simulink model "sil_test"  (R2022b)
settings: Solver=VariableStepAuto  StartTime=0.0  StopTime=inf  RelTol=1e-3
undefined symbols (not defined in the file): battery_monitor, battery_monitor_lib, BM_STATUSES, canChannel, DI_STATUSES, driver_interface, driver_interface_lib, Ended, governor, governor_lib, MI_STATUSES, motor_interface, motor_interface_lib, simp_vd_interface, simp_vd_lib, Single
libraries: canmsglib x16, canlib x10, simulink x6, speedgoatlib_IO191 x5, slrealtimeiplib x3, AMK_comms_plant_lib x1, BMS_plant_lib x1, speedgoatlib_IO614 x1, slrealtimeutilitieslib x1, etargetslib x1
(part 2 of 3)

== system sil_test/Function-Call Subsystem ==
  In1 : Inport
  function : TriggerPort  TriggerType=function-call  VariantControl=(inherit)
  Bus Creator : BusCreator  Inputs=2
  Bus Creator1 : BusCreator  Inputs=7
  Bus Creator2 : BusCreator  Inputs=7
  CAN Unpack : canmsglib/CAN Unpack  CANdbFile=C:\Users\LinF\Documents\MACFE\Embedded\CAN_Stuff\CAN_Databases\CAN_AMKInverter.dbc  MsgList=AMK0_SetPoints1  MsgName=AMK0_SetPoints1  MsgIDType=Standard (11-bit identifier)  MsgIdentifier=389  MsgLength=8  SignalInfo={'AMK_TargetVelocity','16','16','LE','signed','Standard','0','1','0','-Inf','Inf';'AMK_TorqueLimitNegativ','48','16','LE','signed','Standard','0','1','0','-Inf','Inf';'AMK_TorqueLimitPositiv','32','16','LE','signed','Standard','0','1','0','-Inf','Inf';'AMK_bDcOn','9','1','LE','unsigned','Standard','0','1','0','-Inf','Inf';'AMK_bEnable','10','1','LE','unsigned','Standard','0','1','0','-Inf','Inf';'AMK_bErrorReset','11','1','LE','unsigned','Standard','0','1','0','-Inf','Inf';'AMK_bInverterOn','8','1','LE','unsigned','Standard','0','1','0','-Inf','Inf'}  IDPort=off  TimestampPort=off  ErrorPort=off  RemotePort=off  LengthPort=off  StatusPort=off  ApplyMinMax=off
      settings: LibrarySourceBlock=canlib/CAN Unpack  DataFormat=CANdb specified signals
  CAN Unpack1 : canmsglib/CAN Unpack  CANdbFile=C:\Users\LinF\Documents\MACFE\Embedded\CAN_Stuff\CAN_Databases\CAN_AMKInverter.dbc  MsgList=AMK1_SetPoints1  MsgName=AMK1_SetPoints1  MsgIDType=Standard (11-bit identifier)  MsgIdentifier=390  MsgLength=8  SignalInfo={'AMK_TargetVelocity','16','16','LE','signed','Standard','0','1','0','-Inf','Inf';'AMK_TorqueLimitNegativ','48','16','LE','signed','Standard','0','1','0','-Inf','Inf';'AMK_TorqueLimitPositiv','32','16','LE','signed','Standard','0','1','0','-Inf','Inf';'AMK_bDcOn','9','1','LE','unsigned','Standard','0','1','0','-Inf','Inf';'AMK_bEnable','10','1','LE','unsigned','Standard','0','1','0','-Inf','Inf';'AMK_bErrorReset','11','1','LE','unsigned','Standard','0','1','0','-Inf','Inf';'AMK_bInverterOn','8','1','LE','unsigned','Standard','0','1','0','-Inf','Inf'}  IDPort=off  TimestampPort=off  ErrorPort=off  RemotePort=off  LengthPort=off  StatusPort=off  ApplyMinMax=off
      settings: LibrarySourceBlock=canlib/CAN Unpack  DataFormat=CANdb specified signals
  pt_CAN_IN : Outport
  wires:
  Bus Creator/1 -> pt_CAN_IN/1
  Bus Creator2/1 -> Bus Creator/2  "ptCAN_AMK1_Setpoints1_Right"
  Bus Creator1/1 -> Bus Creator/1  "ptCAN_AMK0_Setpoints1_Left"
  In1/1 -> CAN Unpack/1, CAN Unpack1/1
  CAN Unpack/1 -> Bus Creator1/1  "AMK0_TargetVelocity"
  CAN Unpack/2 -> Bus Creator1/2  "AMK0_TorqueLimitNegativ"
  CAN Unpack/3 -> Bus Creator1/3  "AMK0_TorqueLimitPositiv"
  CAN Unpack/4 -> Bus Creator1/4  "AMK0_bDcOn"
  CAN Unpack/5 -> Bus Creator1/5  "AMK0_bEnable"
  CAN Unpack/6 -> Bus Creator1/6  "AMK0_bErrorReset"
  CAN Unpack/7 -> Bus Creator1/7  "AMK0_bInverterOn"
  CAN Unpack1/3 -> Bus Creator2/3  "AMK1_TorqueLimitPositiv"
  CAN Unpack1/6 -> Bus Creator2/6  "AMK1_bErrorReset"
  CAN Unpack1/4 -> Bus Creator2/4  "AMK1_bDcOn"
  CAN Unpack1/7 -> Bus Creator2/7  "AMK1_bInverterOn"
  CAN Unpack1/2 -> Bus Creator2/2  "AMK1_TorqueLimitNegativ"
  CAN Unpack1/5 -> Bus Creator2/5  "AMK1_bEnable"
  CAN Unpack1/1 -> Bus Creator2/1  "AMK1_TargetVelocity"

== system sil_test/Function-Call Subsystem1 ==
  In1 : Inport
  function : TriggerPort  TriggerType=function-call  VariantControl=(inherit)
  Bus Creator1 : BusCreator  Inputs=3
  CAN Unpack : canmsglib/CAN Unpack  CANdbFile=C:\Users\LinF\Documents\MACFE\Controls\repos\can_dbc\dbcs\VEH_CAN.dbc  MsgList=Contactor_States  MsgName=Contactor_States  MsgIDType=Standard (11-bit identifier)  MsgIdentifier=1570  MsgLength=3  SignalInfo={'Pack_Negative','16','8','LE','unsigned','Standard','0','1','0','-Inf','Inf';'Pack_Positive','0','8','LE','unsigned','Standard','0','1','0','-Inf','Inf';'Pack_Precharge','8','8','LE','unsigned','Standard','0','1','0','-Inf','Inf'}  IDPort=off  TimestampPort=off  ErrorPort=off  RemotePort=off  LengthPort=off  StatusPort=off  ApplyMinMax=off
      settings: LibrarySourceBlock=canlib/CAN Unpack  DataFormat=CANdb specified signals
  pt_CAN_IN : Outport
  wires:
  Bus Creator1/1 -> pt_CAN_IN/1  "ptCAN_AMK_Setpoints1_Left"
  In1/1 -> CAN Unpack/1
  CAN Unpack/3 -> Bus Creator1/3  "precharge"
  CAN Unpack/1 -> Bus Creator1/1  "AIR_neg"
  CAN Unpack/2 -> Bus Creator1/2  "AIR_pos"

== system sil_test/Function-Call Subsystem2 ==
  In1 : Inport
  function : TriggerPort  TriggerType=function-call  VariantControl=(inherit)
  CAN Unpack : canmsglib/CAN Unpack  CANdbFile=C:\Users\maxfa\OneDrive\Documents\vehicle_control_system\src\testing\Vehicle_HIL_plant\VEH_CAN.dbc  MsgList=Contactor_Feedback  MsgName=Contactor_Feedback  MsgIDType=Standard (11-bit identifier)  MsgIdentifier=1574  MsgLength=3  SignalInfo={'Pack_Negative_Feedback','8','1','LE','unsigned','Standard','0','1','0','0','1';'Pack_Positive_Feedback','0','1','LE','unsigned','Standard','0','1','0','0','1';'Pack_Precharge_Feedback','16','1','LE','unsigned','Standard','0','1','0','0','1'}  IDPort=off  TimestampPort=off  ErrorPort=off  RemotePort=off  LengthPort=off  StatusPort=off  ApplyMinMax=off
      settings: LibrarySourceBlock=canlib/CAN Unpack  DataFormat=CANdb specified signals
  BM_b_prechrgContactorSts : Outport
  BM_b_HVposContactorSts : Outport  Port=2
  BM_b_HVnegContactorSts : Outport  Port=3
  wires:
  In1/1 -> CAN Unpack/1
  CAN Unpack/1 -> BM_b_HVnegContactorSts/1
  CAN Unpack/3 -> BM_b_prechrgContactorSts/1
  CAN Unpack/2 -> BM_b_HVposContactorSts/1

== system sil_test/Speedgoat Inputs ==
  "Analog input " : speedgoatlib_IO191/Analog input   parModuleId=1  parSampleTime=-1  parPciSlot=-1  parAdcChannels=[1 2 3 4 5 6 7 8]  parAdcMode=2  parAdcRanges=[4 4 4 4 4 4 4 4]  parAdcInitValues=[0 0]  parAdcResets=[1 1]  paramsAdcDma=[0 1 200 -1]
      settings: SourceProductName=Simulink Real-Time: Speedgoat I/O Blockset
  Bus Creator : BusCreator  Inputs=16
  "Digital input " : speedgoatlib_IO191/Digital input   parModuleId=1  parSampleTime=-1  parPciSlot=-1  parDiChannels=[1 2 3 4 5 6 7 8]
      settings: SourceProductName=Simulink Real-Time: Speedgoat I/O Blockset
  Speedgoat Inputs : Outport
  inverter_en : Outport  Port=2
  wires:
  Bus Creator/1 -> Speedgoat Inputs/1
  "Digital input "/1 -> inverter_en/1, Bus Creator/1  "DIO1"
  "Digital input "/2 -> Bus Creator/2  "DIO2"
  "Digital input "/3 -> Bus Creator/3  "DIO3"
  "Digital input "/4 -> Bus Creator/4  "DIO4"
  "Digital input "/5 -> Bus Creator/5  "DIO5"
  "Digital input "/6 -> Bus Creator/6  "DIO6"
  "Digital input "/7 -> Bus Creator/7  "DIO7"
  "Digital input "/8 -> Bus Creator/8  "DIO8"
  "Analog input "/1 -> Bus Creator/9  "AI1"
  "Analog input "/2 -> Bus Creator/10  "AI2"
  "Analog input "/3 -> Bus Creator/11  "AI3"
  "Analog input "/4 -> Bus Creator/12  "AI4"
  "Analog input "/5 -> Bus Creator/13  "AI5"
  "Analog input "/6 -> Bus Creator/14  "AI6"
  "Analog input "/7 -> Bus Creator/15  "AI7"
  "Analog input "/8 -> Bus Creator/16  "AI8"

== system sil_test/Speedgoat Outputs ==
  Speedgoat Outputs : Inport
  "Analog output " : speedgoatlib_IO191/Analog output   parModuleId=1  parSampleTime=-1  parPciSlot=-1  parDacChannels=[1 2 3 4]  parModuleType=1  parDacRanges=[3 3 3 3]  parDacInitValues=[0 0 0 0]  parDacResets=[1 1 1 1]
      settings: SourceProductName=Simulink Real-Time: Speedgoat I/O Blockset
  Bus Selector : BusSelector  OutputSignals=DO9,DO10,DO11,DO12,DO13,DO14,DO15,DO16,AO1,AO2,AO3,AO4
  "Digital output " : speedgoatlib_IO191/Digital output   parModuleId=1  parSampleTime=-1  parPciSlot=-1  parDoChannels=[9 10 11 12 13 14 15 16]  parDoInitValues=[0 0 0 0 0 0 0 0]  parDoResets=[1 1 1 1 1 1 1 1]
      settings: SourceProductName=Simulink Real-Time: Speedgoat I/O Blockset
  wires:
  Speedgoat Outputs/1 -> Bus Selector/1
  Bus Selector/4 -> "Digital output "/4  "<DO12>"
  Bus Selector/1 -> "Digital output "/1  "<DO9>"
  Bus Selector/2 -> "Digital output "/2  "<DO10>"
  Bus Selector/5 -> "Digital output "/5  "<DO13>"
  Bus Selector/3 -> "Digital output "/3  "<DO11>"
  Bus Selector/6 -> "Digital output "/6  "<DO14>"
  Bus Selector/7 -> "Digital output "/7  "<DO15>"
  Bus Selector/8 -> "Digital output "/8  "<DO16>"
  Bus Selector/9 -> "Analog output "/1  "<AO1>"
  Bus Selector/10 -> "Analog output "/2  "<AO2>"
  Bus Selector/11 -> "Analog output "/3  "<AO3>"
  Bus Selector/12 -> "Analog output "/4  "<AO4>"

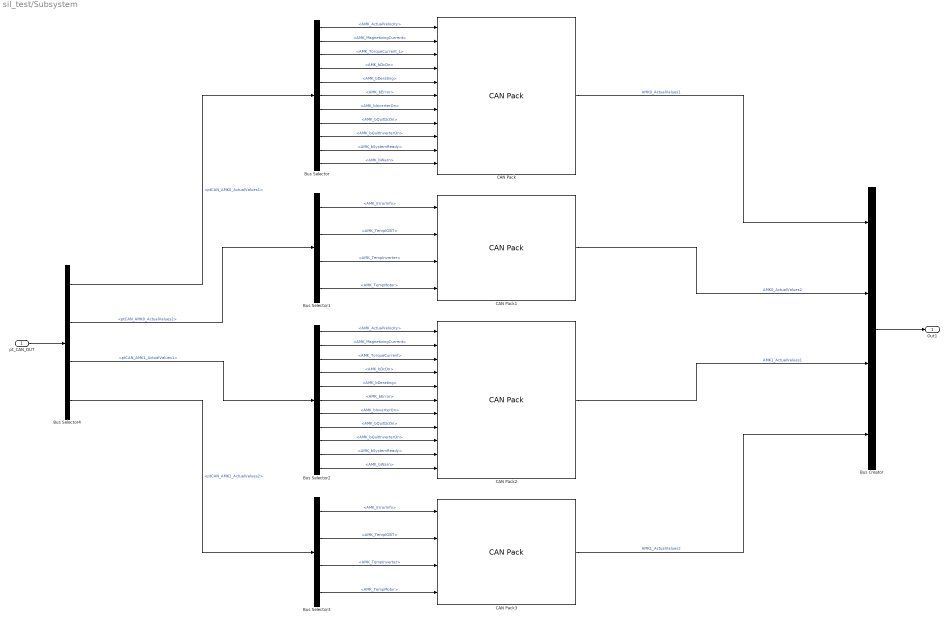
== system sil_test/Subsystem ==
  pt_CAN_OUT : Inport
  Bus Creator : BusCreator  Inputs=4
  Bus Selector : BusSelector  OutputSignals=AMK_ActualVelocity,AMK_MagnetizingCurrent,AMK_TorqueCurrent_L,AMK_bDcOn,AMK_bDerating,AMK_bError,AMK_bInverterOn,AMK_bQuitDcOn,AMK_bQuitInverterOn,AMK_bSystemReady,AMK_bWarn
  Bus Selector1 : BusSelector  OutputSignals=AMK_ErrorInfo,AMK_TempIGBT,AMK_TempInverter,AMK_TempMotor
  Bus Selector2 : BusSelector  OutputSignals=AMK_ActualVelocity,AMK_MagnetizingCurrent,AMK_TorqueCurrent,AMK_bDcOn,AMK_bDerating,AMK_bError,AMK_bInverterOn,AMK_bQuitDcOn,AMK_bQuitInverterOn,AMK_bSystemReady,AMK_bWarn
  Bus Selector3 : BusSelector  OutputSignals=AMK_ErrorInfo,AMK_TempIGBT,AMK_TempInverter,AMK_TempMotor
  Bus Selector4 : BusSelector  OutputSignals=ptCAN_AMK0_ActualValues1,ptCAN_AMK0_ActualValues2,ptCAN_AMK1_ActualValues1,ptCAN_AMK1_ActualValues2
  CAN Pack : canmsglib/CAN Pack  CANdbFile=C:\Users\LinF\Documents\MACFE\Embedded\CAN_Stuff\CAN_Databases\CAN_AMKInverter.dbc  MsgList=AMK0_ActualValues1  MsgName=AMK0_ActualValues1  MsgIDType=Standard (11-bit identifier)  MsgIdentifier=644  MsgLength=8  Remote=off  ApplyMinMax=off  BusOutput=off  SignalInfo={'AMK_ActualVelocity','16','16','LE','signed','Standard','0','1','0','-Inf','Inf';'AMK_MagnetizingCurrent','48','16','LE','signed','Standard','0','1','0','-Inf','Inf';'AMK_TorqueCurrent','32','16','LE','signed','Standard','0','1','0','-Inf','Inf';'AMK_bDcOn','12','1','LE','unsigned','Standard','0','1','0','-Inf','Inf';'AMK_bDerating','15','1','LE','unsigned','Standard','0','1','0','-Inf','Inf';'AMK_bError','9','1','LE','unsigned','Standard','0','1','0','-Inf','Inf';'AMK_bInverterOn','14','1','LE','unsigned','Standard','0','1','0','-Inf','Inf';'AMK_bQuitDcOn','11','1','LE','unsigned','Standard','0','1','0','-Inf','Inf';'AMK_bQuitInverterOn','13','1','LE','unsigned','Standard','0','1','0','-Inf','Inf';'AMK_bSystemReady','8','1','LE','unsigned','Standard','0','1','0','-Inf','Inf';'AMK_bWarn','10','1','LE','unsigned','Standard','0','1','0','-Inf','Inf'}
      settings: LibrarySourceBlock=canlib/CAN Pack  DataFormat=CANdb specified signals
  CAN Pack1 : canmsglib/CAN Pack  CANdbFile=C:\Users\LinF\Documents\MACFE\Embedded\CAN_Stuff\CAN_Databases\CAN_AMKInverter.dbc  MsgList=AMK0_ActualValues2  MsgName=AMK0_ActualValues2  MsgIDType=Standard (11-bit identifier)  MsgIdentifier=646  MsgLength=8  Remote=off  ApplyMinMax=off  BusOutput=off  SignalInfo={'AMK_ErrorInfo','32','16','LE','unsigned','Standard','0','1','0','0','65535';'AMK_TempIGBT','48','16','LE','signed','Standard','0','0.1','0','-3276.8','3276.7';'AMK_TempInverter','16','16','LE','signed','Standard','0','0.1','0','-3276.8','3276.7';'AMK_TempMotor','0','16','LE','signed','Standard','0','0.1','0','-3276.8','3276.7'}
      settings: LibrarySourceBlock=canlib/CAN Pack  DataFormat=CANdb specified signals
  CAN Pack2 : canmsglib/CAN Pack  CANdbFile=C:\Users\LinF\Documents\MACFE\Embedded\CAN_Stuff\CAN_Databases\CAN_AMKInverter.dbc  MsgList=AMK1_ActualValues1  MsgName=AMK1_ActualValues1  MsgIDType=Standard (11-bit identifier)  MsgIdentifier=645  MsgLength=8  Remote=off  ApplyMinMax=off  BusOutput=off  SignalInfo={'AMK_ActualVelocity','16','16','LE','signed','Standard','0','1','0','-Inf','Inf';'AMK_MagnetizingCurrent','48','16','LE','signed','Standard','0','1','0','-Inf','Inf';'AMK_TorqueCurrent','32','16','LE','signed','Standard','0','1','0','-Inf','Inf';'AMK_bDcOn','12','1','LE','unsigned','Standard','0','1','0','-Inf','Inf';'AMK_bDerating','15','1','LE','unsigned','Standard','0','1','0','-Inf','Inf';'AMK_bError','9','1','LE','unsigned','Standard','0','1','0','-Inf','Inf';'AMK_bInverterOn','14','1','LE','unsigned','Standard','0','1','0','-Inf','Inf';'AMK_bQuitDcOn','11','1','LE','unsigned','Standard','0','1','0','-Inf','Inf';'AMK_bQuitInverterOn','13','1','LE','unsigned','Standard','0','1','0','-Inf','Inf';'AMK_bSystemReady','8','1','LE','unsigned','Standard','0','1','0','-Inf','Inf';'AMK_bWarn','10','1','LE','unsigned','Standard','0','1','0','-Inf','Inf'}
      settings: LibrarySourceBlock=canlib/CAN Pack  DataFormat=CANdb specified signals
  CAN Pack3 : canmsglib/CAN Pack  CANdbFile=C:\Users\LinF\Documents\MACFE\Embedded\CAN_Stuff\CAN_Databases\CAN_AMKInverter.dbc  MsgList=AMK1_ActualValues2  MsgName=AMK1_ActualValues2  MsgIDType=Standard (11-bit identifier)  MsgIdentifier=647  MsgLength=8  Remote=off  ApplyMinMax=off  BusOutput=off  SignalInfo={'AMK_ErrorInfo','32','16','LE','unsigned','Standard','0','1','0','0','65535';'AMK_TempIGBT','48','16','LE','signed','Standard','0','0.1','0','-3276.8','3276.7';'AMK_TempInverter','16','16','LE','signed','Standard','0','0.1','0','-3276.8','3276.7';'AMK_TempMotor','0','16','LE','signed','Standard','0','0.1','0','-3276.8','3276.7'}
      settings: LibrarySourceBlock=canlib/CAN Pack  DataFormat=CANdb specified signals
  Out1 : Outport
  wires:
  CAN Pack/1 -> Bus Creator/1  "AMK0_ActualValues1"
  CAN Pack1/1 -> Bus Creator/2  "AMK0_ActualValues2"
  CAN Pack2/1 -> Bus Creator/3  "AMK1_ActualValues1"
  CAN Pack3/1 -> Bus Creator/4  "AMK1_ActualValues2"
  Bus Selector4/1 -> Bus Selector/1  "<ptCAN_AMK0_ActualValues1>"
  Bus Selector4/2 -> Bus Selector1/1  "<ptCAN_AMK0_ActualValues2>"
  Bus Selector4/3 -> Bus Selector2/1  "<ptCAN_AMK1_ActualValues1>"
  Bus Selector4/4 -> Bus Selector3/1  "<ptCAN_AMK1_ActualValues2>"
  pt_CAN_OUT/1 -> Bus Selector4/1
  Bus Creator/1 -> Out1/1
  Bus Selector/1 -> CAN Pack/1  "<AMK_ActualVelocity>"
  Bus Selector/3 -> CAN Pack/3  "<AMK_TorqueCurrent_L>"
  Bus Selector/2 -> CAN Pack/2  "<AMK_MagnetizingCurrent>"
  Bus Selector/4 -> CAN Pack/4  "<AMK_bDcOn>"
  Bus Selector/5 -> CAN Pack/5  "<AMK_bDerating>"
  Bus Selector/6 -> CAN Pack/6  "<AMK_bError>"
  Bus Selector/7 -> CAN Pack/7  "<AMK_bInverterOn>"
  Bus Selector/8 -> CAN Pack/8  "<AMK_bQuitDcOn>"
  Bus Selector/9 -> CAN Pack/9  "<AMK_bQuitInverterOn>"
  Bus Selector/10 -> CAN Pack/10  "<AMK_bSystemReady>"
  Bus Selector/11 -> CAN Pack/11  "<AMK_bWarn>"
  Bus Selector1/1 -> CAN Pack1/1  "<AMK_ErrorInfo>"
  Bus Selector1/2 -> CAN Pack1/2  "<AMK_TempIGBT>"
  Bus Selector1/3 -> CAN Pack1/3  "<AMK_TempInverter>"
  Bus Selector1/4 -> CAN Pack1/4  "<AMK_TempMotor>"
  Bus Selector2/3 -> CAN Pack2/3  "<AMK_TorqueCurrent>"
  Bus Selector3/1 -> CAN Pack3/1  "<AMK_ErrorInfo>"
  Bus Selector2/7 -> CAN Pack2/7  "<AMK_bInverterOn>"
  Bus Selector2/4 -> CAN Pack2/4  "<AMK_bDcOn>"
  Bus Selector2/2 -> CAN Pack2/2  "<AMK_MagnetizingCurrent>"
  Bus Selector3/4 -> CAN Pack3/4  "<AMK_TempMotor>"
  Bus Selector3/2 -> CAN Pack3/2  "<AMK_TempIGBT>"
  Bus Selector2/5 -> CAN Pack2/5  "<AMK_bDerating>"
  Bus Selector2/10 -> CAN Pack2/10  "<AMK_bSystemReady>"
  Bus Selector3/3 -> CAN Pack3/3  "<AMK_TempInverter>"
  Bus Selector2/8 -> CAN Pack2/8  "<AMK_bQuitDcOn>"
  Bus Selector2/6 -> CAN Pack2/6  "<AMK_bError>"
  Bus Selector2/11 -> CAN Pack2/11  "<AMK_bWarn>"
  Bus Selector2/1 -> CAN Pack2/1  "<AMK_ActualVelocity>"
  Bus Selector2/9 -> CAN Pack2/9  "<AMK_bQuitInverterOn>"

== system sil_test/Subsystem1 ==
  pt_CAN_OUT : Inport
  Bus Selector4 : BusSelector  OutputSignals=AIR_neg_sts,AIR_pos_sts,precharge_sts
  CAN Pack : canmsglib/CAN Pack  CANdbFile=C:\Users\LinF\Documents\MACFE\Controls\repos\can_dbc\dbcs\VEH_CAN.dbc  MsgList=Contactor_Feedback  MsgName=Contactor_Feedback  MsgIDType=Standard (11-bit identifier)  MsgIdentifier=1574  MsgLength=3  Remote=off  ApplyMinMax=off  BusOutput=off  SignalInfo={'Pack_Negative_Feedback','8','1','LE','unsigned','Standard','0','1','0','0','1';'Pack_Positive_Feedback','0','1','LE','unsigned','Standard','0','1','0','0','1';'Pack_Precharge_Feedback','16','1','LE','unsigned','Standard','0','1','0','0','1'}
      settings: LibrarySourceBlock=canlib/CAN Pack  DataFormat=CANdb specified signals
  Out1 : Outport
  wires:
  pt_CAN_OUT/1 -> Bus Selector4/1
  Bus Selector4/2 -> CAN Pack/2  "<AIR_pos_sts>"
  Bus Selector4/3 -> CAN Pack/3  "<precharge_sts>"
  Bus Selector4/1 -> CAN Pack/1  "<AIR_neg_sts>"
  CAN Pack/1 -> Out1/1

== system sil_test/TCP Server ==
  Speedgoat Inputs : Inport
  Bus Creator : BusCreator  Inputs=12
  Bus Selector : BusSelector  OutputSignals=DIO1,DIO2,DIO3,DIO4,DIO5,DIO6,DIO7,DIO8,AI1,AI2,AI3,AI4,AI5,AI6,AI7,AI8
  Constant : Constant
  Receive : Subsystem
  Send : Subsystem
  Setup : Subsystem
  Speedgoat Outputs : Outport
  wires:
  Constant/1 -> Setup/1(Enable Server)
  Setup/1(Server Status) -> Send/17(Enable), Receive/1(Enable)
  Receive/1(DO9) -> Bus Creator/1  "DO9"
  Receive/2(DO10) -> Bus Creator/2  "DO10"
  Receive/3(DO11) -> Bus Creator/3  "DO11"
  Receive/4(DO12) -> Bus Creator/4  "DO12"
  Receive/5(DO13) -> Bus Creator/5  "DO13"
  Receive/6(DO14) -> Bus Creator/6  "DO14"
  Receive/7(DO15) -> Bus Creator/7  "DO15"
  Receive/8(DO16) -> Bus Creator/8  "DO16"
  Receive/9(AO1) -> Bus Creator/9  "AO1"
  Receive/10(AO2) -> Bus Creator/10  "AO2"
  Receive/11(AO3) -> Bus Creator/11  "AO3"
  Receive/12(AO4) -> Bus Creator/12  "AO4"
  Bus Creator/1 -> Speedgoat Outputs/1
  Speedgoat Inputs/1 -> Bus Selector/1
  Bus Selector/1 -> Send/1(DI1)  "<DIO1>"
  Bus Selector/2 -> Send/2(DI2)  "<DIO2>"
  Bus Selector/3 -> Send/3(DI3)  "<DIO3>"
  Bus Selector/4 -> Send/4(DI4)  "<DIO4>"
  Bus Selector/5 -> Send/5(DI5)  "<DIO5>"
  Bus Selector/6 -> Send/6(DI6)  "<DIO6>"
  Bus Selector/7 -> Send/7(DI7)  "<DIO7>"
  Bus Selector/8 -> Send/8(DI8)  "<DIO8>"
  Bus Selector/9 -> Send/9(AI1)  "<AI1>"
  Bus Selector/10 -> Send/10(AI2)  "<AI2>"
  Bus Selector/11 -> Send/11(AI3)  "<AI3>"
  Bus Selector/12 -> Send/12(AI4)  "<AI4>"
  Bus Selector/13 -> Send/13(AI5)  "<AI5>"
  Bus Selector/14 -> Send/14(AI6)  "<AI6>"
  Bus Selector/15 -> Send/15(AI7)  "<AI7>"
  Bus Selector/16 -> Send/16(AI8)  "<AI8>"

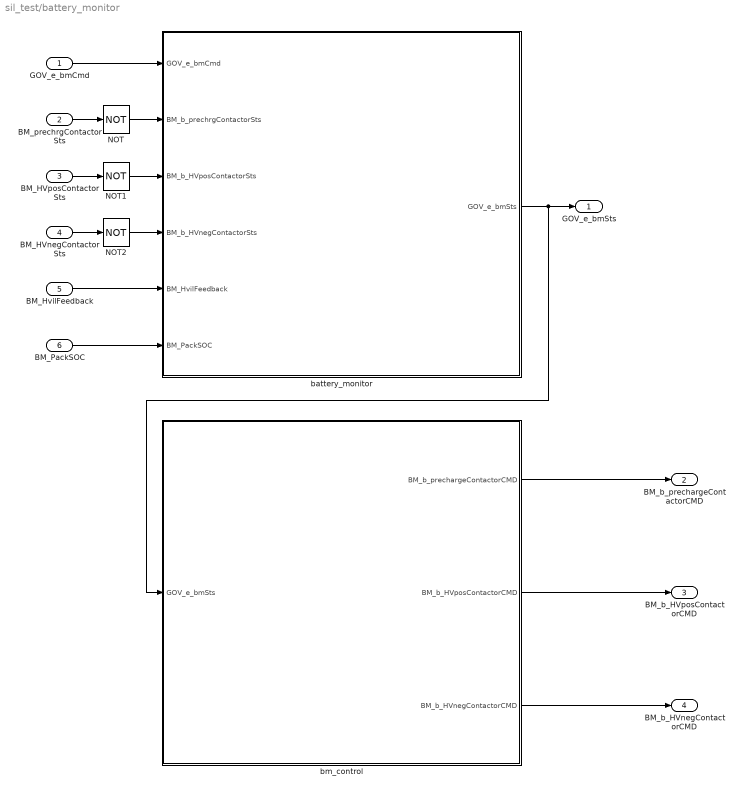
== system sil_test/battery_monitor ==
  GOV_e_bmCmd : Inport
  BM_prechrgContactorSts : Inport  Port=2
  BM_HVposContactorSts : Inport  Port=3
  BM_HVnegContactorSts : Inport  Port=4
  BM_HvilFeedback : Inport  Port=5
  BM_PackSOC : Inport  Port=6
  NOT : Logic  Operator=NOT  IconShape=distinctive  AllPortsSameDT=off  OutDataTypeStr=boolean
  NOT1 : Logic  Operator=NOT  IconShape=distinctive  AllPortsSameDT=off  OutDataTypeStr=boolean
  NOT2 : Logic  Operator=NOT  IconShape=distinctive  AllPortsSameDT=off  OutDataTypeStr=boolean
  battery_monitor : Stateflow chart  TreatAsAtomicUnit=on
  bm_control : Stateflow chart  TreatAsAtomicUnit=on
  GOV_e_bmSts : Outport
  BM_b_prechargeContactorCMD : Outport  Port=2
  BM_b_HVposContactorCMD : Outport  Port=3
  BM_b_HVnegContactorCMD : Outport  Port=4
  wires:
  NOT2/1 -> battery_monitor/4(BM_b_HVnegContactorSts)
  NOT1/1 -> battery_monitor/3(BM_b_HVposContactorSts)
  NOT/1 -> battery_monitor/2(BM_b_prechrgContactorSts)
  bm_control/3(BM_b_HVnegContactorCMD) -> BM_b_HVnegContactorCMD/1
  bm_control/1(BM_b_prechargeContactorCMD) -> BM_b_prechargeContactorCMD/1
  bm_control/2(BM_b_HVposContactorCMD) -> BM_b_HVposContactorCMD/1
  battery_monitor/1(GOV_e_bmSts) -> GOV_e_bmSts/1, bm_control/1(GOV_e_bmSts)
  BM_HVnegContactorSts/1 -> NOT2/1
  BM_HVposContactorSts/1 -> NOT1/1
  BM_prechrgContactorSts/1 -> NOT/1
  GOV_e_bmCmd/1 -> battery_monitor/1(GOV_e_bmCmd)
  BM_HvilFeedback/1 -> battery_monitor/5(BM_HvilFeedback)
  BM_PackSOC/1 -> battery_monitor/6(BM_PackSOC)

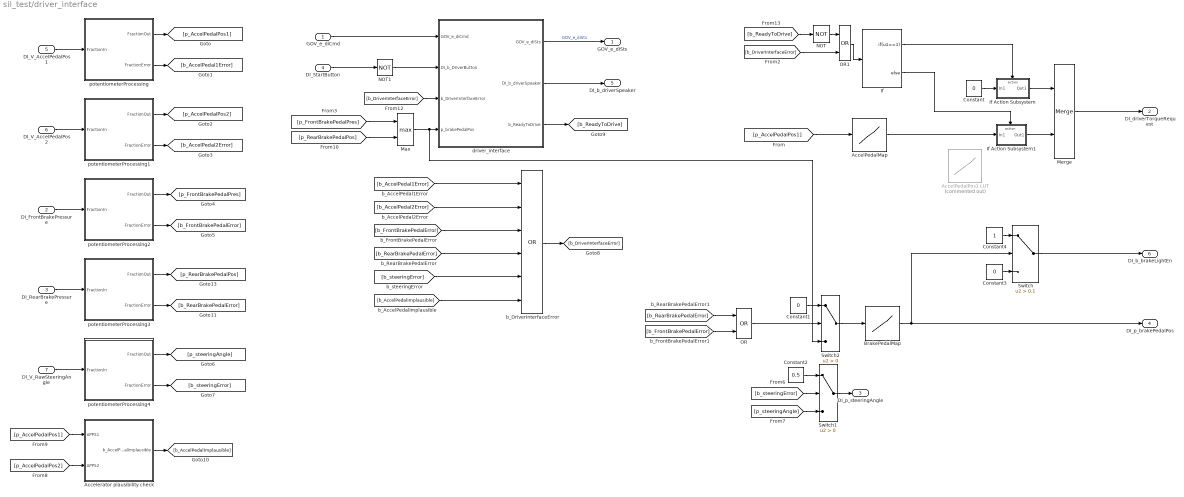
== system sil_test/driver_interface ==
  GOV_e_diCmd : Inport
  DI_FrontBrakePressure : Inport  Port=2
  DI_RearBrakePressure : Inport  Port=3
  DI_StartButton : Inport  Port=4
  DI_V_AccelPedalPos1 : Inport  Port=5
  DI_V_AccelPedalPos2 : Inport  Port=6
  Dl_V_RawSteeringAngle : Inport  Port=7
  AccelPedalMap : Lookup_n-D  NumberOfTableDimensions=1  BreakpointsForDimension1=[0 1]  Table=[0 1]  ExtrapMethod=Clip  InternalRulePriority=Speed  RndMeth=Simplest
  AccelPedalPos1 LUT : Lookup_n-D  Commented=on  NumberOfTableDimensions=1  BreakpointsForDimension1=[0 1 2 3 4 5 6 7 8 9 10 11 12 13 14 15 16 17 18 19 20 21 22 23 24 25 26 27 28 29 30 31 32 33 34 35 36 37 38 39 40 41 42 43 44 45 46 47 48 49 50 51 52 53 54 55 56 57 58 59 60 61 62 63 64 65 66 67 68 69 70 71 72 73 74 75 76 77 78 79 80 81 82 83 84 85 86 87 88 89 90 91 92 93 94 95 96 97 98 99]  Table=[0 0 0 0 0 0 0 0 0 0 0 0 0 0 0 0 0 0 0 0 0 0 1.85185185185185 3.7037037037037 5.55555555555556 7.40740740740741 9.25925925925926 11.1111111111111 12.962962962963 14.8148148148148 16.6666666666667 18.5185185185185 20.3703703703704 22.2222222222222 24.0740740740741 25.9259259259259 27.7777777777778 29.6296296296296 31.4814814814815 33.3333333333333 35.1851851851852 37.037037037037 38.8888888888889 40.7407407407407 42.5925925925926 44.4444444444444 46.2962962962963 48.1481481481481 50 51.8518518518519 53.7037037037037 55.5555555555556 57.4074074074074 59.2592592592593 61.1111111111111 62.962962962963 64.8148148148148 66.6666666666667 68.5185185185185 70.3703703703704 72.2222222222222 74.0740740740741 75.9259259259259 77.7777777777778 79.6296296296296 81.4814814814815 83.3333333333333 85.1851851851852 87.037037037037 88.8888888888889 90.7407407407407 92.5925925925926 94.4444444444444 96.2962962962963 98.1481481481482 100 100 100 100 100 100 100 100 100 100 100 100 100 100 100 100 100 100 100 100 100 100 100 100 100]  ExtrapMethod=Clip  InternalRulePriority=Speed  RndMeth=Simplest
  Accelerator plausibility check : Subsystem
  BrakePedalMap : Lookup_n-D  NumberOfTableDimensions=1  BreakpointsForDimension1=[0 5 10 15 20 25 30 35 40 45 50 55 60 65 70 75 80 85 90 95 100]  Table=[0 5 10 15 20 25 30 35 40 45 50 55 60 65 70 75 80 85 90 95 100]  ExtrapMethod=Clip  InternalRulePriority=Speed  RndMeth=Simplest
  Constant : Constant  Value=0  OutDataTypeStr=double
  Constant1 : Constant  Value=0  OutDataTypeStr=single
  Constant2 : Constant  Value=0.5  OutDataTypeStr=single
  Constant3 : Constant  Value=0  OutDataTypeStr=boolean
  Constant4 : Constant  OutDataTypeStr=boolean
  If : If  IfExpression=u1==1
  If Action Subsystem : Subsystem  TreatAsAtomicUnit=on
  If Action Subsystem1 : Subsystem  TreatAsAtomicUnit=on
  Max : MinMax  Function=max  Inputs=2
  Merge : Merge
  NOT : Logic  Operator=NOT  IconShape=distinctive  AllPortsSameDT=off  OutDataTypeStr=boolean
  NOT1 : Logic  Operator=NOT  IconShape=distinctive  AllPortsSameDT=off  OutDataTypeStr=boolean
  OR : Logic  Operator=OR  AllPortsSameDT=off  OutDataTypeStr=boolean
  OR1 : Logic  Operator=OR  AllPortsSameDT=off  OutDataTypeStr=boolean
  Switch : Switch  Criteria=u2 > Threshold  Threshold=0.1  SaturateOnIntegerOverflow=off  InputSameDT=off
  Switch1 : Switch  Criteria=u2 > Threshold  SaturateOnIntegerOverflow=off  InputSameDT=off
  Switch2 : Switch  Criteria=u2 > Threshold  SaturateOnIntegerOverflow=off  InputSameDT=off
  b_DriverInterfaceError : Logic  Operator=OR  Inputs=6  AllPortsSameDT=off  OutDataTypeStr=boolean
  driver_interface : Stateflow chart  TreatAsAtomicUnit=on
  potentiometerProcessing : Subsystem
  potentiometerProcessing1 : Subsystem
  potentiometerProcessing2 : Subsystem
  potentiometerProcessing3 : Subsystem
  potentiometerProcessing4 : Subsystem
  GOV_e_diSts : Outport
  DI_driverTorqueRequest : Outport  Port=2
  DI_p_steeringAngle : Outport  Port=3
  DI_p_brakePedalPos : Outport  Port=4
  DI_b_driverSpeaker : Outport  Port=5
  DI_b_brakeLightEn : Outport  Port=6
  wires:
  DI_StartButton/1 -> NOT1/1
  GOV_e_diCmd/1 -> driver_interface/1(GOV_e_diCmd)
  NOT1/1 -> driver_interface/2(DI_b_DriverButton)
  BrakePedalMap/1 -> Switch/2, DI_p_brakePedalPos/1
  [p_FrontBrakePedalPres] -> Max/1
  Dl_V_RawSteeringAngle/1 -> potentiometerProcessing4/1(FractionIn)
  DI_V_AccelPedalPos2/1 -> potentiometerProcessing1/1(FractionIn)
  b_DriverInterfaceError/1 -> [b_DriverInterfaceError]
  NOT/1 -> OR1/1
  [b_ReadyToDrive] -> NOT/1
  [b_DriverInterfaceError] -> OR1/2
  OR1/1 -> If/1
  driver_interface/3(b_ReadyToDrive) -> [b_ReadyToDrive]
  If/2 -> If Action Subsystem1/Action
  Constant/1 -> If Action Subsystem/1(In1)
  driver_interface/2(DI_b_driverSpeaker) -> DI_b_driverSpeaker/1
  [b_DriverInterfaceError] -> driver_interface/3(b_DriverInterfaceError)
  [b_steeringError] -> b_DriverInterfaceError/5
  [b_FrontBrakePedalError] -> b_DriverInterfaceError/3
  [b_AccelPedal1Error] -> b_DriverInterfaceError/1
  [b_AccelPedal2Error] -> b_DriverInterfaceError/2
  [p_steeringAngle] -> Switch1/3
  [b_steeringError] -> Switch1/2
  Switch1/1 -> DI_p_steeringAngle/1
  Constant2/1 -> Switch1/1
  Switch2/1 -> BrakePedalMap/1
  Max/1 -> Switch2/3, driver_interface/4(p_brakePedalPos)
  Constant1/1 -> Switch2/1
  If Action Subsystem1/1(Out1) -> Merge/2
  If/1 -> If Action Subsystem/Action
  If Action Subsystem/1(Out1) -> Merge/1
  potentiometerProcessing4/2(FractionError) -> [b_steeringError]
  potentiometerProcessing4/1(FractionOut) -> [p_steeringAngle]
  potentiometerProcessing2/1(FractionOut) -> [p_FrontBrakePedalPres]
  potentiometerProcessing2/2(FractionError) -> [b_FrontBrakePedalError]
  potentiometerProcessing1/2(FractionError) -> [b_AccelPedal2Error]
  potentiometerProcessing1/1(FractionOut) -> [p_AccelPedalPos2]
  potentiometerProcessing/2(FractionError) -> [b_AccelPedal1Error]
  potentiometerProcessing/1(FractionOut) -> [p_AccelPedalPos1]
  DI_V_AccelPedalPos1/1 -> potentiometerProcessing/1(FractionIn)
  Merge/1 -> DI_driverTorqueRequest/1
  driver_interface/1(GOV_e_diSts) -> GOV_e_diSts/1  "GOV_e_diSts"
  Switch/1 -> DI_b_brakeLightEn/1
  [p_AccelPedalPos1] -> Accelerator plausibility check/1(APPS1)
  [p_AccelPedalPos2] -> Accelerator plausibility check/2(APPS2)
  Accelerator plausibility check/1(b_AccelPedalImplausible) -> [b_AccelPedalImplausible]
  [b_AccelPedalImplausible] -> b_DriverInterfaceError/6
  DI_FrontBrakePressure/1 -> potentiometerProcessing2/1(FractionIn)
  DI_RearBrakePressure/1 -> potentiometerProcessing3/1(FractionIn)
  potentiometerProcessing3/2(FractionError) -> [b_RearBrakePedalError]
  [b_RearBrakePedalError] -> b_DriverInterfaceError/4
  potentiometerProcessing3/1(FractionOut) -> [p_RearBrakePedalPos]
  [p_RearBrakePedalPos] -> Max/2
  [b_FrontBrakePedalError] -> OR/2
  [b_RearBrakePedalError] -> OR/1
  OR/1 -> Switch2/2
  [p_AccelPedalPos1] -> AccelPedalMap/1
  AccelPedalMap/1 -> If Action Subsystem1/1(In1)
  Constant3/1 -> Switch/3
  Constant4/1 -> Switch/1

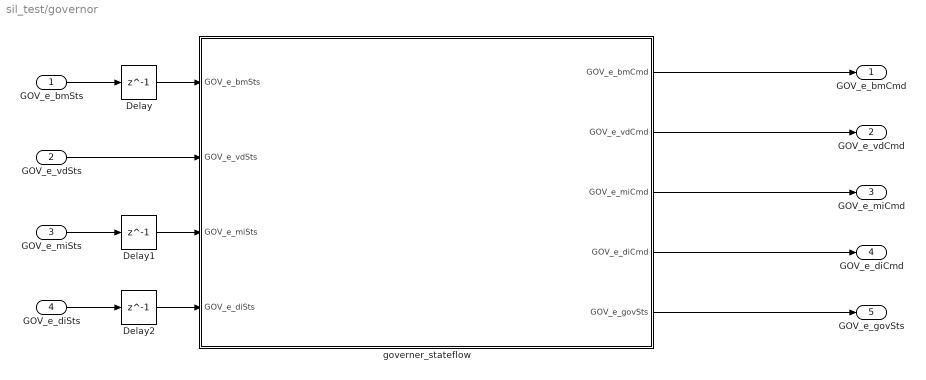
== system sil_test/governor ==
  GOV_e_bmSts : Inport
  GOV_e_vdSts : Inport  Port=2
  GOV_e_miSts : Inport  Port=3
  GOV_e_diSts : Inport  Port=4
  Delay : Delay  DelayLength=1  InitialCondition=BM_STATUSES.BM_UNKNOWN
  Delay1 : Delay  DelayLength=1  InitialCondition=MI_STATUSES.UNKNOWN
  Delay2 : Delay  DelayLength=1  InitialCondition=DI_STATUSES.DI_UNKNOWN
  governer_stateflow : Stateflow chart  TreatAsAtomicUnit=on
  GOV_e_bmCmd : Outport
  GOV_e_vdCmd : Outport  Port=2
  GOV_e_miCmd : Outport  Port=3
  GOV_e_diCmd : Outport  Port=4
  GOV_e_govSts : Outport  Port=5
  wires:
  Delay2/1 -> governer_stateflow/4(GOV_e_diSts)
  Delay1/1 -> governer_stateflow/3(GOV_e_miSts)
  Delay/1 -> governer_stateflow/1(GOV_e_bmSts)
  GOV_e_miSts/1 -> Delay1/1
  governer_stateflow/4(GOV_e_diCmd) -> GOV_e_diCmd/1
  governer_stateflow/3(GOV_e_miCmd) -> GOV_e_miCmd/1
  governer_stateflow/2(GOV_e_vdCmd) -> GOV_e_vdCmd/1
  governer_stateflow/1(GOV_e_bmCmd) -> GOV_e_bmCmd/1
  GOV_e_diSts/1 -> Delay2/1
  GOV_e_vdSts/1 -> governer_stateflow/2(GOV_e_vdSts)
  GOV_e_bmSts/1 -> Delay/1
  governer_stateflow/5(GOV_e_govSts) -> GOV_e_govSts/1

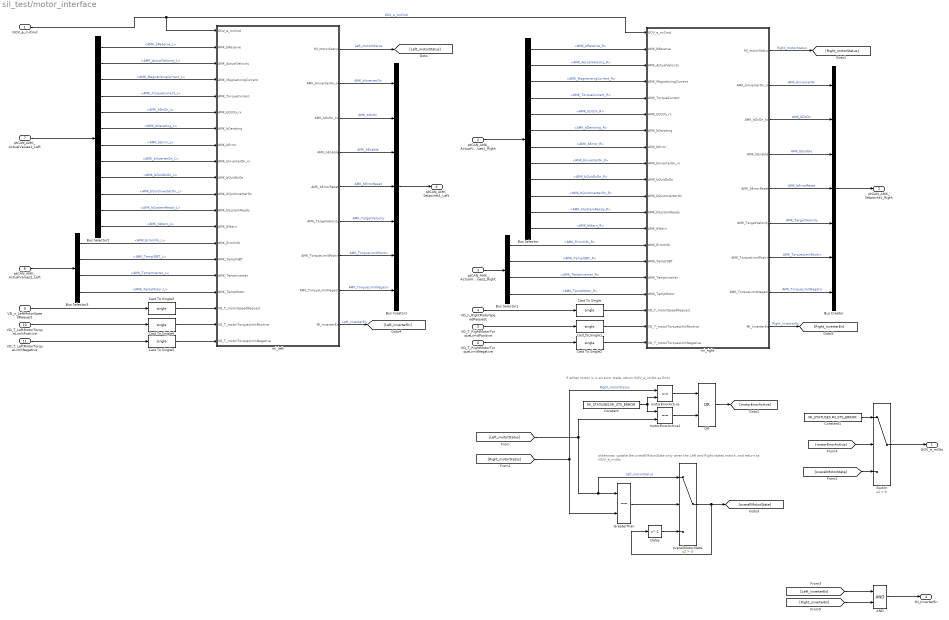
== system sil_test/motor_interface ==
  note: if either motor is in an error state, return GOV_e_miSts as Error
  note: otherwise, update the overallMotorState only when the Left and Right states match, and return as GOV_e_miSts
  GOV_e_miCmd : Inport
  ptCAN_AMK_ActualValues1_Right : Inport  Port=2
  ptCAN_AMK_ActualValues2_Right : Inport  Port=3
  VD_n_RightMotorSpeedRequest : Inport  Port=4
  VD_T_RightMotorTorqueLimitPositive : Inport  Port=5
  VD_T_RightMotorTorqueLimitNegative : Inport  Port=6
  ptCAN_AMK_ActualValues1_Left : Inport  Port=7
  ptCAN_AMK_ActualValues2_Left : Inport  Port=8
  VD_n_LeftMotorSpeedRequest : Inport  Port=9
  VD_T_LeftMotorTorqueLimitPositive : Inport  Port=10
  VD_T_LeftMotorTorqueLimitNegative : Inport  Port=11
  AND : Logic  AllPortsSameDT=off  OutDataTypeStr=boolean
  Bus Creator : BusCreator  Inputs=7
  Bus Creator1 : BusCreator  Inputs=7
  Bus Selector : BusSelector  OutputSignals=AMK_bReserve_R,AMK_ActualVelocity_R,AMK_MagnetizingCurrent_R,AMK_TorqueCurrent_R,AMK_bDcOn_R,AMK_bDerating_R,AMK_bError_R,AMK_bInverterOn_R,AMK_bQuitDcOn_R,AMK_bQuitInverterOn_R,AMK_bSystemReady_R,AMK_bWarn_R
  Bus Selector1 : BusSelector  OutputSignals=AMK_ErrorInfo_R,AMK_TempIGBT_R,AMK_TempInverter_R,AMK_TempMotor_R
  Bus Selector2 : BusSelector  OutputSignals=AMK_bReserve_L,AMK_ActualVelocity_L,AMK_MagnetizingCurrent_L,AMK_TorqueCurrent_L,AMK_bDcOn_L,AMK_bDerating_L,AMK_bError_L,AMK_bInverterOn_L,AMK_bQuitDcOn_L,AMK_bQuitInverterOn_L,AMK_bSystemReady_L,AMK_bWarn_L
  Bus Selector3 : BusSelector  OutputSignals=AMK_ErrorInfo_L,AMK_TempIGBT_L,AMK_TempInverter_L,AMK_TempMotor_L
  Cast To Single{,1..5} (6 alike) : DataTypeConversion  OutDataTypeStr=single  SaturateOnIntegerOverflow=off  RndMeth=Floor
  Constant : Constant  Value=MI_STATUSES.MI_STS_ERROR  OutDataTypeStr=Enum: MI_STATUSES
  Constant1 : Constant  Value=MI_STATUSES.MI_STS_ERROR  OutDataTypeStr=Enum: MI_STATUSES
  Delay : Delay  DelayLength=1  InitialCondition=MI_STATUSES.OFF
  GreaterThan : RelationalOperator  Operator===  OutDataTypeStr=boolean  RndMeth=Simplest  InputSameDT=off
  OR : Logic  Operator=OR  IconShape=distinctive  AllPortsSameDT=off  OutDataTypeStr=boolean
  Switch : Switch  Criteria=u2 > Threshold  SaturateOnIntegerOverflow=off  InputSameDT=off
  mi_left : Stateflow chart  TreatAsAtomicUnit=on
  mi_right : Stateflow chart  TreatAsAtomicUnit=on
  motorErrorActive : RelationalOperator  Operator===  OutDataTypeStr=boolean  RndMeth=Simplest  InputSameDT=off
  motorErrorActive1 : RelationalOperator  Operator===  OutDataTypeStr=boolean  RndMeth=Simplest  InputSameDT=off
  overallMotorState : Switch  Criteria=u2 > Threshold  SaturateOnIntegerOverflow=off  InputSameDT=off
  GOV_e_miSts : Outport
  ptCAN_AMK_Setpoints1_Right : Outport  Port=2
  ptCAN_AMK_Setpoints1_Left : Outport  Port=3
  MI_InverterEn : Outport  Port=4
  wires:
  ptCAN_AMK_ActualValues2_Left/1 -> Bus Selector3/1
  Bus Creator1/1 -> ptCAN_AMK_Setpoints1_Left/1
  mi_left/2(AMK_bInverterOn_tx) -> Bus Creator1/1  "AMK_bInverterOn"
  mi_left/4(AMK_bEnable) -> Bus Creator1/3  "AMK_bEnable"
  mi_left/6(AMK_TargetVelocity) -> Bus Creator1/5  "AMK_TargetVelocity"
  mi_left/3(AMK_bDcOn_tx) -> Bus Creator1/2  "AMK_bDcOn"
  mi_left/5(AMK_bErrorReset) -> Bus Creator1/4  "AMK_bErrorReset"
  mi_left/7(AMK_TorqueLimitPositiv) -> Bus Creator1/6  "AMK_TorqueLimitPositiv"
  mi_left/8(AMK_TorqueLimitNegativ) -> Bus Creator1/7  "AMK_TorqueLimitNegativ"
  ptCAN_AMK_ActualValues1_Left/1 -> Bus Selector2/1
  Bus Selector2/1 -> mi_left/2(AMK_bReserve)  "<AMK_bReserve_L>"
  VD_T_LeftMotorTorqueLimitPositive/1 -> Cast To Single4/1
  VD_T_LeftMotorTorqueLimitNegative/1 -> Cast To Single5/1
  VD_n_LeftMotorSpeedRequest/1 -> Cast To Single3/1
  VD_n_RightMotorSpeedRequest/1 -> Cast To Single/1
  VD_T_RightMotorTorqueLimitNegative/1 -> Cast To Single2/1
  VD_T_RightMotorTorqueLimitPositive/1 -> Cast To Single1/1
  mi_right/8(AMK_TorqueLimitNegativ) -> Bus Creator/7  "AMK_TorqueLimitNegativ"
  mi_right/7(AMK_TorqueLimitPositiv) -> Bus Creator/6  "AMK_TorqueLimitPositiv"
  Constant1/1 -> Switch/1
  motorErrorActive/1 -> OR/1
  motorErrorActive1/1 -> OR/2
  OR/1 -> [motorErrorActive]
  [overallMotorState] -> Switch/3
  GreaterThan/1 -> overallMotorState/2
  Delay/1 -> overallMotorState/3
  overallMotorState/1 -> [overallMotorState], Delay/1
  [motorErrorActive] -> Switch/2
  Switch/1 -> GOV_e_miSts/1
  Constant/1 -> motorErrorActive1/1, motorErrorActive/2
  [Right_motorStatus] -> GreaterThan/2, motorErrorActive/1  "Right_motorStatus"
  [Left_motorStatus] -> GreaterThan/1, overallMotorState/1, motorErrorActive1/2  "Left_motorStatus"
  mi_right/1(MI_motorStatus) -> [Right_motorStatus]  "Right_motorStatus"
  mi_left/1(MI_motorStatus) -> [Left_motorStatus]  "Left_motorStatus"
  mi_right/5(AMK_bErrorReset) -> Bus Creator/4  "AMK_bErrorReset"
  mi_right/3(AMK_bDcOn_tx) -> Bus Creator/2  "AMK_bDcOn"
  mi_right/6(AMK_TargetVelocity) -> Bus Creator/5  "AMK_TargetVelocity"
  mi_right/4(AMK_bEnable) -> Bus Creator/3  "AMK_bEnable"
  mi_right/2(AMK_bInverterOn_tx) -> Bus Creator/1  "AMK_bInverterOn"
  Bus Creator/1 -> ptCAN_AMK_Setpoints1_Right/1
  Bus Selector1/4 -> mi_right/17(AMK_TempMotor)  "<AMK_TempMotor_R>"
  Bus Selector1/3 -> mi_right/16(AMK_TempInverter)  "<AMK_TempInverter_R>"
  Bus Selector1/2 -> mi_right/15(AMK_TempIGBT)  "<AMK_TempIGBT_R>"
  Bus Selector1/1 -> mi_right/14(AMK_ErrorInfo)  "<AMK_ErrorInfo_R>"
  ptCAN_AMK_ActualValues2_Right/1 -> Bus Selector1/1
  Bus Selector/1 -> mi_right/2(AMK_bReserve)  "<AMK_bReserve_R>"
  Bus Selector/12 -> mi_right/13(AMK_bWarn)  "<AMK_bWarn_R>"
  Bus Selector/11 -> mi_right/12(AMK_bSystemReady)  "<AMK_bSystemReady_R>"
  Bus Selector/10 -> mi_right/11(AMK_bQuitInverterOn)  "<AMK_bQuitInverterOn_R>"
  Bus Selector/9 -> mi_right/10(AMK_bQuitDcOn)  "<AMK_bQuitDcOn_R>"
  Bus Selector/8 -> mi_right/9(AMK_bInverterOn_rx)  "<AMK_bInverterOn_R>"
  Bus Selector/7 -> mi_right/8(AMK_bError)  "<AMK_bError_R>"
  Bus Selector/6 -> mi_right/7(AMK_bDerating)  "<AMK_bDerating_R>"
  Bus Selector/5 -> mi_right/6(AMK_bDcOn_rx)  "<AMK_bDcOn_R>"
  Bus Selector/4 -> mi_right/5(AMK_TorqueCurrent)  "<AMK_TorqueCurrent_R>"
  Bus Selector/3 -> mi_right/4(AMK_MagnetizingCurrent)  "<AMK_MagnetizingCurrent_R>"
  Bus Selector/2 -> mi_right/3(AMK_ActualVelocity)  "<AMK_ActualVelocity_R>"
  ptCAN_AMK_ActualValues1_Right/1 -> Bus Selector/1
  GOV_e_miCmd/1 -> mi_right/1(GOV_e_miCmd), mi_left/1(GOV_e_miCmd)  "GOV_e_miCmd"
  Cast To Single/1 -> mi_right/18(VD_T_motorSpeedRequest)
  Cast To Single1/1 -> mi_right/19(VD_T_motorTorqueLimitPositive)
  Cast To Single2/1 -> mi_right/20(VD_T_motorTorqueLimitNegative)
  Cast To Single3/1 -> mi_left/18(VD_T_motorSpeedRequest)
  Cast To Single4/1 -> mi_left/19(VD_T_motorTorqueLimitPositive)
  Cast To Single5/1 -> mi_left/20(VD_T_motorTorqueLimitNegative)
  Bus Selector2/2 -> mi_left/3(AMK_ActualVelocity)  "<AMK_ActualVelocity_L>"
  Bus Selector2/3 -> mi_left/4(AMK_MagnetizingCurrent)  "<AMK_MagnetizingCurrent_L>"
  Bus Selector2/4 -> mi_left/5(AMK_TorqueCurrent)  "<AMK_TorqueCurrent_L>"
  Bus Selector2/5 -> mi_left/6(AMK_bDcOn_rx)  "<AMK_bDcOn_L>"
  Bus Selector2/6 -> mi_left/7(AMK_bDerating)  "<AMK_bDerating_L>"
  Bus Selector2/7 -> mi_left/8(AMK_bError)  "<AMK_bError_L>"
  Bus Selector2/8 -> mi_left/9(AMK_bInverterOn_rx)  "<AMK_bInverterOn_L>"
  Bus Selector2/9 -> mi_left/10(AMK_bQuitDcOn)  "<AMK_bQuitDcOn_L>"
  Bus Selector2/10 -> mi_left/11(AMK_bQuitInverterOn)  "<AMK_bQuitInverterOn_L>"
  Bus Selector2/11 -> mi_left/12(AMK_bSystemReady)  "<AMK_bSystemReady_L>"
  Bus Selector2/12 -> mi_left/13(AMK_bWarn)  "<AMK_bWarn_L>"
  Bus Selector3/1 -> mi_left/14(AMK_ErrorInfo)  "<AMK_ErrorInfo_L>"
  Bus Selector3/2 -> mi_left/15(AMK_TempIGBT)  "<AMK_TempIGBT_L>"
  Bus Selector3/3 -> mi_left/16(AMK_TempInverter)  "<AMK_TempInverter_L>"
  Bus Selector3/4 -> mi_left/17(AMK_TempMotor)  "<AMK_TempMotor_L>"
  AND/1 -> MI_InverterEn/1
  mi_left/9(MI_InverterEn) -> [Left_inverterEn]  "Left_inverterEn"
  mi_right/9(MI_InverterEn) -> [Right_inverterEn]  "Right_inverterEn"
  [Left_inverterEn] -> AND/1
  [Right_inverterEn] -> AND/2

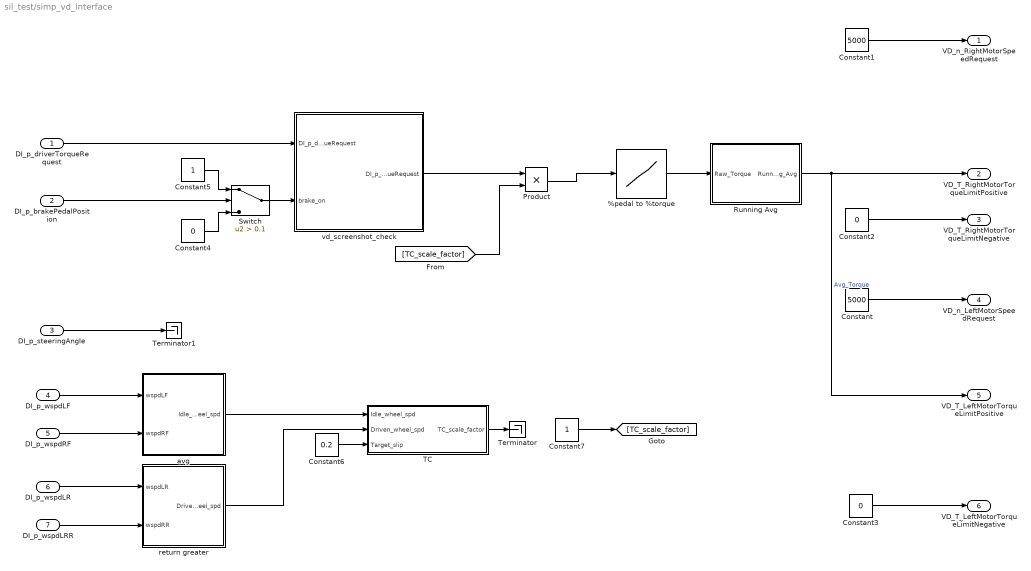
== system sil_test/simp_vd_interface ==
  DI_p_driverTorqueRequest : Inport
  DI_p_brakePedalPosition : Inport  Port=2
  DI_p_steeringAngle : Inport  Port=3
  DI_p_wspdLF : Inport  Port=4
  DI_p_wspdRF : Inport  Port=5
  DI_p_wspdLR : Inport  Port=6
  DI_p_wspdLRR : Inport  Port=7
  %pedal to %torque : Lookup_n-D  NumberOfTableDimensions=1  BreakpointsForDimension1=[linspace(0,1,101)]  Table=[linspace(0,1000,101)]  InternalRulePriority=Speed  RndMeth=Simplest
  Constant : Constant  Value=5000
  Constant1 : Constant  Value=5000
  Constant2 : Constant  Value=0
  Constant3 : Constant  Value=0
  Constant4 : Constant  Value=0
  Constant5 : Constant
  Constant6 : Constant  Value=0.2
  Constant7 : Constant
  Product : Product
  Running Avg : Subsystem
  Switch : Switch  Criteria=u2 > Threshold  Threshold=0.1  SaturateOnIntegerOverflow=off  InputSameDT=off
  TC : Subsystem
  Terminator : Terminator
  Terminator1 : Terminator
  avg : MATLAB Function  TreatAsAtomicUnit=on
  return greater : MATLAB Function  TreatAsAtomicUnit=on
  vd_screenshot_check : Stateflow chart  TreatAsAtomicUnit=on
  VD_n_RightMotorSpeedRequest : Outport
  VD_T_RightMotorTorqueLimitPositive : Outport  Port=2
  VD_T_RightMotorTorqueLimitNegative : Outport  Port=3
  VD_n_LeftMotorSpeedRequest : Outport  Port=4
  VD_T_LeftMotorTorqueLimitPositive : Outport  Port=5
  VD_T_LeftMotorTorqueLimitNegative : Outport  Port=6
  wires:
  [TC_scale_factor] -> Product/2
  Product/1 -> %pedal to %torque/1
  Constant6/1 -> TC/3(Target_slip)
  return greater/1(Driven_wheel_spd) -> TC/2(Driven_wheel_spd)
  DI_p_wspdLRR/1 -> return greater/2(wspdRR)
  DI_p_wspdLR/1 -> return greater/1(wspdLR)
  avg/1(Idle_wheel_spd) -> TC/1(Idle_wheel_spd)
  DI_p_wspdRF/1 -> avg/2(wspdRF)
  DI_p_wspdLF/1 -> avg/1(wspdLF)
  DI_p_steeringAngle/1 -> Terminator1/1
  Constant/1 -> VD_n_LeftMotorSpeedRequest/1
  Constant1/1 -> VD_n_RightMotorSpeedRequest/1
  Constant2/1 -> VD_T_RightMotorTorqueLimitNegative/1
  Constant3/1 -> VD_T_LeftMotorTorqueLimitNegative/1
  Constant4/1 -> Switch/3
  Constant5/1 -> Switch/1
  Switch/1 -> vd_screenshot_check/2(brake_on)
  DI_p_brakePedalPosition/1 -> Switch/2
  DI_p_driverTorqueRequest/1 -> vd_screenshot_check/1(DI_p_driverTorqueRequest)
  %pedal to %torque/1 -> Running Avg/1(Raw_Torque)
  Running Avg/1(Running_Avg) -> VD_T_LeftMotorTorqueLimitPositive/1, VD_T_RightMotorTorqueLimitPositive/1  "Avg_Torque"
  vd_screenshot_check/1(DI_p_motorTorqueRequest) -> Product/1
  TC/1(TC_scale_factor) -> Terminator/1
  Constant7/1 -> [TC_scale_factor]

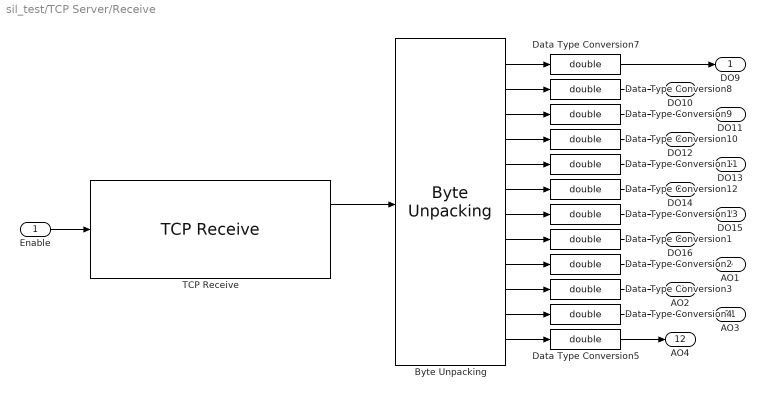
== system sil_test/TCP Server/Receive ==
  Enable : Inport
  Byte Unpacking : slrealtimeutilitieslib/Byte Unpacking  MaskUnpackedDataTypes={'uint8','uint8','uint8','uint8','uint8','uint8','uint8','uint8','double','double','double','double'}  MaskUnpackedDataSizes={1,1,1,1,1,1,1,1,1,1,1,1}  MaskAlignment=1
  Data Type Conversion{1..5,7..13} (12 alike) : DataTypeConversion  OutDataTypeStr=double  SaturateOnIntegerOverflow=off  RndMeth=Floor
  TCP Receive : slrealtimeiplib/TCP Receive  socketAddPortVal=Server: 192.168.10.1:8001  rcvWidth=40  sampleTime=0.01
  DO9 : Outport
  DO10 : Outport  Port=2
  DO11 : Outport  Port=3
  DO12 : Outport  Port=4
  DO13 : Outport  Port=5
  DO14 : Outport  Port=6
  DO15 : Outport  Port=7
  DO16 : Outport  Port=8
  AO1 : Outport  Port=9
  AO2 : Outport  Port=10
  AO3 : Outport  Port=11
  AO4 : Outport  Port=12
  wires:
  Enable/1 -> TCP Receive/1
  TCP Receive/1 -> Byte Unpacking/1
  Byte Unpacking/8 -> Data Type Conversion1/1
  Byte Unpacking/7 -> Data Type Conversion13/1
  Byte Unpacking/2 -> Data Type Conversion8/1
  Byte Unpacking/6 -> Data Type Conversion12/1
  Data Type Conversion8/1 -> DO10/1
  Data Type Conversion10/1 -> DO12/1
  Data Type Conversion9/1 -> DO11/1
  Byte Unpacking/5 -> Data Type Conversion11/1
  Byte Unpacking/1 -> Data Type Conversion7/1
  Byte Unpacking/3 -> Data Type Conversion9/1
  Data Type Conversion12/1 -> DO14/1
  Byte Unpacking/10 -> Data Type Conversion3/1
  Byte Unpacking/9 -> Data Type Conversion2/1
  Byte Unpacking/4 -> Data Type Conversion10/1
  Data Type Conversion13/1 -> DO15/1
  Data Type Conversion11/1 -> DO13/1
  Byte Unpacking/12 -> Data Type Conversion5/1
  Data Type Conversion7/1 -> DO9/1
  Byte Unpacking/11 -> Data Type Conversion4/1
  Data Type Conversion1/1 -> DO16/1
  Data Type Conversion2/1 -> AO1/1
  Data Type Conversion3/1 -> AO2/1
  Data Type Conversion4/1 -> AO3/1
  Data Type Conversion5/1 -> AO4/1

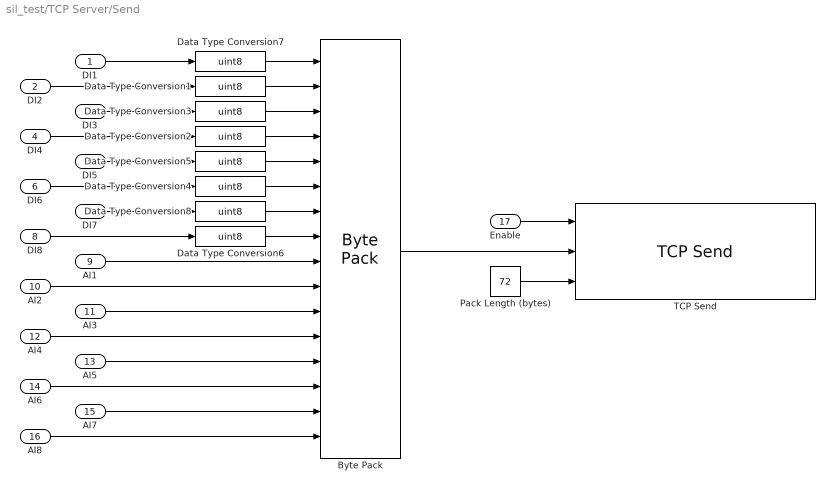
== system sil_test/TCP Server/Send ==
  DI1 : Inport
  DI2 : Inport  Port=2
  DI3 : Inport  Port=3
  DI4 : Inport  Port=4
  DI5 : Inport  Port=5
  DI6 : Inport  Port=6
  DI7 : Inport  Port=7
  DI8 : Inport  Port=8
  AI1 : Inport  Port=9
  AI2 : Inport  Port=10
  AI3 : Inport  Port=11
  AI4 : Inport  Port=12
  AI5 : Inport  Port=13
  AI6 : Inport  Port=14
  AI7 : Inport  Port=15
  AI8 : Inport  Port=16
  Enable : Inport  Port=17
  Byte Pack : etargetslib/Byte Pack  datatypes={'uint8','uint8','uint8','uint8','uint8','uint8','uint8','uint8','double','double','double','double','double','double','double','double'}  byteAlign=1
  Data Type Conversion{1..8} (8 alike) : DataTypeConversion  OutDataTypeStr=uint8  SaturateOnIntegerOverflow=off  RndMeth=Floor
  Pack Length (bytes) : Constant  Value=72
  TCP Send : slrealtimeiplib/TCP Send  socketAddPortVal=Server: 192.168.10.1:8001  sampleTime=0.01
  wires:
  Enable/1 -> TCP Send/1
  DI1/1 -> Data Type Conversion7/1
  DI2/1 -> Data Type Conversion1/1
  DI3/1 -> Data Type Conversion3/1
  DI4/1 -> Data Type Conversion2/1
  DI5/1 -> Data Type Conversion5/1
  DI6/1 -> Data Type Conversion4/1
  DI7/1 -> Data Type Conversion8/1
  DI8/1 -> Data Type Conversion6/1
  AI1/1 -> Byte Pack/9
  AI2/1 -> Byte Pack/10
  AI3/1 -> Byte Pack/11
  AI4/1 -> Byte Pack/12
  Byte Pack/1 -> TCP Send/2
  Data Type Conversion7/1 -> Byte Pack/1
  Data Type Conversion1/1 -> Byte Pack/2
  Data Type Conversion3/1 -> Byte Pack/3
  Data Type Conversion2/1 -> Byte Pack/4
  Data Type Conversion4/1 -> Byte Pack/6
  Data Type Conversion5/1 -> Byte Pack/5
  Data Type Conversion6/1 -> Byte Pack/8
  Data Type Conversion8/1 -> Byte Pack/7
  AI5/1 -> Byte Pack/13
  AI6/1 -> Byte Pack/14
  AI7/1 -> Byte Pack/15
  AI8/1 -> Byte Pack/16
  Pack Length (bytes)/1 -> TCP Send/3

== system sil_test/TCP Server/Setup ==
  Enable Server : Inport
  "Setup " : speedgoatlib_IO191/Setup   parModuleId=1  parPciSlot=-1  parTriggerSignal=TTL  parAdcChannels=[1 2 3 4 5 6 7 8]  parAdcRanges=[4 4 4 4 4 4 4 4]  parAdcChannel1=on  parAdcChannel2=on  parAdcChannel3=on  parAdcChannel4=on  parAdcChannel5=on  parAdcChannel6=on  parAdcChannel7=on  parAdcChannel8=on  parAdcMode=Single-Ended  parAdcRange11=+-5.12 V  parAdcRange21=+-24.576 V  parAdcRange12=+-5.12 V  parAdcRange22=+-24.576 V  parAdcRange13=+-5.12 V  parAdcRange23=+-24.576 V  parAdcRange14=+-5.12 V  parAdcRange24=+-24.576 V  parAdcRange15=+-5.12 V  parAdcRange25=+-24.576 V  parAdcRange16=+-5.12 V  parAdcRange26=+-24.576 V  parAdcRange17=+-5.12 V  parAdcRange27=+-24.576 V  parAdcRange18=+-5.12 V  parAdcRange28=+-24.576 V  parAdcEnDma=off  parAdcFrame=125  parAdcDiv=200  parAdcSample=-1  parDacChannels=[1 2 3 4]  parDacChannel1=on  parDacChannel2=on  parDacChannel3=on  parDacChannel4=on  parDacMode=Single-Ended  parDacRanges=[3 3 3 3]  parDacInitValues=[0 0 0 0]  parDacResets=[1 1 1 1]  parDacRange1=+-5 V  parDacInitValue1=0  parDacReset1=on  parDacRange2=+-5 V  parDacInitValue2=0  parDacReset2=on  parDacRange3=+-5 V  parDacInitValue3=0  parDacReset3=on  parDacRange4=+-5 V  parDacInitValue4=0  parDacReset4=on  parDiChannels=[1 2 3 4 5 6 7 8]  parDoChannels=[9 10 11 12 13 14 15 16]  parDioFirstControl=[2 3 4 5 6 7 8 9]  parDioSecondControl=0  parDioChannel1=In  parExtra1=I  parExtra2=I  parExtra3=I  parDioChannel2=Out  parDioChannel3=Out  parDioChannel4=Out  parDioChannel5=Out  parDioChannel6=Out  parDioChannel7=Out  parDioChannel8=Out  parDioChannel9=Out  parDoInitValues=[0 0 0 0]  parDoResets=[1 1 1 1]  parDoInitValue1=0  parDoReset1=on  parDoInitValue2=0  parDoReset2=on  parDoInitValue3=0  parDoReset3=on  parDoInitValue4=0  parDoReset4=on  parDoInitValue5=0  parDoReset5=on  parDoInitValue6=0  parDoReset6=on  parDoInitValue7=0  parDoReset7=on  parDoInitValue8=0  parDoReset8=on  parDoInitValue9=0  parDoReset9=on  parDoInitValue10=0  parDoReset10=on  parDoInitValue11=0  parDoReset11=on  parDoInitValue12=0  parDoReset12=on  parDoInitValue13=0  parDoReset13=on  parDoInitValue14=0  parDoReset14=on  parDoInitValue15=0  parDoReset15=on  parDoInitValue16=0  parDoReset16=on
      settings: SourceProductName=Simulink Real-Time: Speedgoat I/O Blockset
  TCP Server : slrealtimeiplib/TCP Server  Priority=-1  useHostTargetConn=off  serverAddress=192.168.10.1  serverPort=8001
  Server Status : Outport
  wires:
  Enable Server/1 -> TCP Server/1
  TCP Server/1 -> Server Status/1

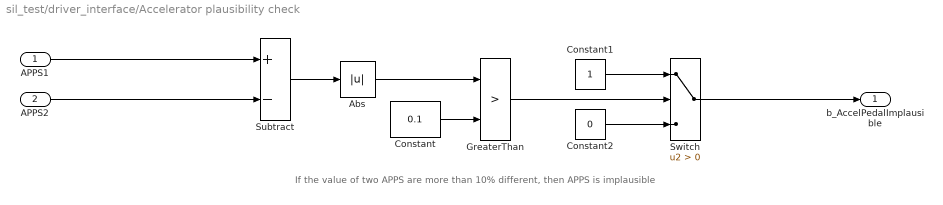
== system sil_test/driver_interface/Accelerator plausibility check ==
  note: If the value of two APPS are more than 10% different, then APPS is implausible
  APPS1 : Inport
  APPS2 : Inport  Port=2
  Abs : Abs  SaturateOnIntegerOverflow=off
  Constant : Constant  Value=0.1
  Constant1 : Constant
  Constant2 : Constant  Value=0
  GreaterThan : RelationalOperator  Operator=>  OutDataTypeStr=boolean  RndMeth=Simplest  InputSameDT=off
  Subtract : Sum  Inputs=+-
  Switch : Switch  Criteria=u2 > Threshold  SaturateOnIntegerOverflow=off  InputSameDT=off
  b_AccelPedalImplausible : Outport
  wires:
  APPS1/1 -> Subtract/1
  APPS2/1 -> Subtract/2
  Subtract/1 -> Abs/1
  Abs/1 -> GreaterThan/1
  Constant/1 -> GreaterThan/2
  GreaterThan/1 -> Switch/2
  Constant1/1 -> Switch/1
  Constant2/1 -> Switch/3
  Switch/1 -> b_AccelPedalImplausible/1

== system sil_test/driver_interface/If Action Subsystem ==
  In1 : Inport
  Action Port : ActionPort  ActionPortLabel=if(u1==1)
  Out1 : Outport
  wires:
  In1/1 -> Out1/1

== system sil_test/driver_interface/If Action Subsystem1 ==
  In1 : Inport
  Action Port : ActionPort  ActionPortLabel=else
  Out1 : Outport
  wires:
  In1/1 -> Out1/1

== system sil_test/driver_interface/potentiometerProcessing ==
  FractionIn : Inport
  Interval Test Dynamic : simulink/Logic and Bit Operations/Interval Test Dynamic  IntervalClosedRight=on  IntervalClosedLeft=on  OutDataTypeStr=boolean
  LowerPotentiometerLimit1 : Constant  Value=0  OutDataTypeStr=double
  NOT : Logic  Operator=NOT  IconShape=distinctive  AllPortsSameDT=off  OutDataTypeStr=boolean
  UpperPotentiometerLimit1 : Constant  OutDataTypeStr=double
  FractionOut : Outport
  FractionError : Outport  Port=2
  wires:
  NOT/1 -> FractionError/1
  FractionIn/1 -> FractionOut/1, Interval Test Dynamic/2
  Interval Test Dynamic/1 -> NOT/1  "withinNominalRange"
  UpperPotentiometerLimit1/1 -> Interval Test Dynamic/1
  LowerPotentiometerLimit1/1 -> Interval Test Dynamic/3

== system sil_test/driver_interface/potentiometerProcessing1 ==
  FractionIn : Inport
  Interval Test Dynamic : simulink/Logic and Bit Operations/Interval Test Dynamic  IntervalClosedRight=on  IntervalClosedLeft=on  OutDataTypeStr=boolean
  LowerPotentiometerLimit1 : Constant  Value=0  OutDataTypeStr=double
  NOT : Logic  Operator=NOT  IconShape=distinctive  AllPortsSameDT=off  OutDataTypeStr=boolean
  UpperPotentiometerLimit1 : Constant  OutDataTypeStr=double
  FractionOut : Outport
  FractionError : Outport  Port=2
  wires:
  NOT/1 -> FractionError/1
  FractionIn/1 -> FractionOut/1, Interval Test Dynamic/2
  Interval Test Dynamic/1 -> NOT/1  "withinNominalRange"
  UpperPotentiometerLimit1/1 -> Interval Test Dynamic/1
  LowerPotentiometerLimit1/1 -> Interval Test Dynamic/3

== system sil_test/driver_interface/potentiometerProcessing2 ==
  FractionIn : Inport
  Interval Test Dynamic : simulink/Logic and Bit Operations/Interval Test Dynamic  IntervalClosedRight=on  IntervalClosedLeft=on  OutDataTypeStr=boolean
  LowerPotentiometerLimit1 : Constant  Value=0  OutDataTypeStr=double
  NOT : Logic  Operator=NOT  IconShape=distinctive  AllPortsSameDT=off  OutDataTypeStr=boolean
  UpperPotentiometerLimit1 : Constant  OutDataTypeStr=double
  FractionOut : Outport
  FractionError : Outport  Port=2
  wires:
  NOT/1 -> FractionError/1
  FractionIn/1 -> FractionOut/1, Interval Test Dynamic/2
  Interval Test Dynamic/1 -> NOT/1  "withinNominalRange"
  UpperPotentiometerLimit1/1 -> Interval Test Dynamic/1
  LowerPotentiometerLimit1/1 -> Interval Test Dynamic/3

== system sil_test/driver_interface/potentiometerProcessing3 ==
  FractionIn : Inport
  Interval Test Dynamic : simulink/Logic and Bit Operations/Interval Test Dynamic  IntervalClosedRight=on  IntervalClosedLeft=on  OutDataTypeStr=boolean
  LowerPotentiometerLimit1 : Constant  Value=0  OutDataTypeStr=double
  NOT : Logic  Operator=NOT  IconShape=distinctive  AllPortsSameDT=off  OutDataTypeStr=boolean
  UpperPotentiometerLimit1 : Constant  OutDataTypeStr=double
  FractionOut : Outport
  FractionError : Outport  Port=2
  wires:
  NOT/1 -> FractionError/1
  FractionIn/1 -> FractionOut/1, Interval Test Dynamic/2
  Interval Test Dynamic/1 -> NOT/1  "withinNominalRange"
  UpperPotentiometerLimit1/1 -> Interval Test Dynamic/1
  LowerPotentiometerLimit1/1 -> Interval Test Dynamic/3
